simulink model "Modelo_global_NL_ley_de_control_minima_eje_d_q"  (R2023b)
settings: Solver=VariableStepAuto  StartTime=0.0  StopTime=1  RelTol=1e-3
values from neighbouring files (symbols this model uses):
  Ld = 6.6e-3    (= 0.0066)    [constantes.m]
  Lq = 5.8e-3    (= 0.0058)    [constantes.m]
  P_p = 3    [constantes.m]
settings Model: Creator=rodri  LastModifiedBy=nahue

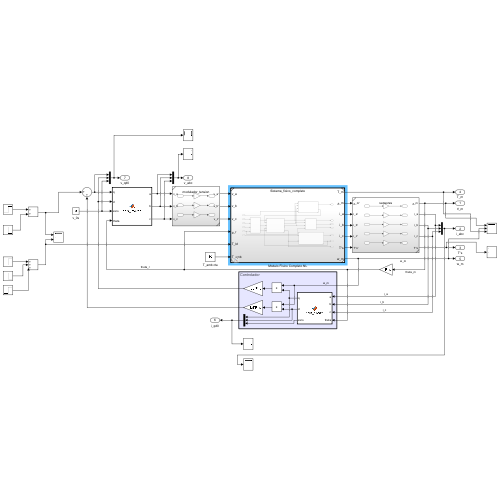
[thumbnail: Simulink's stored preview of the top-level diagram]
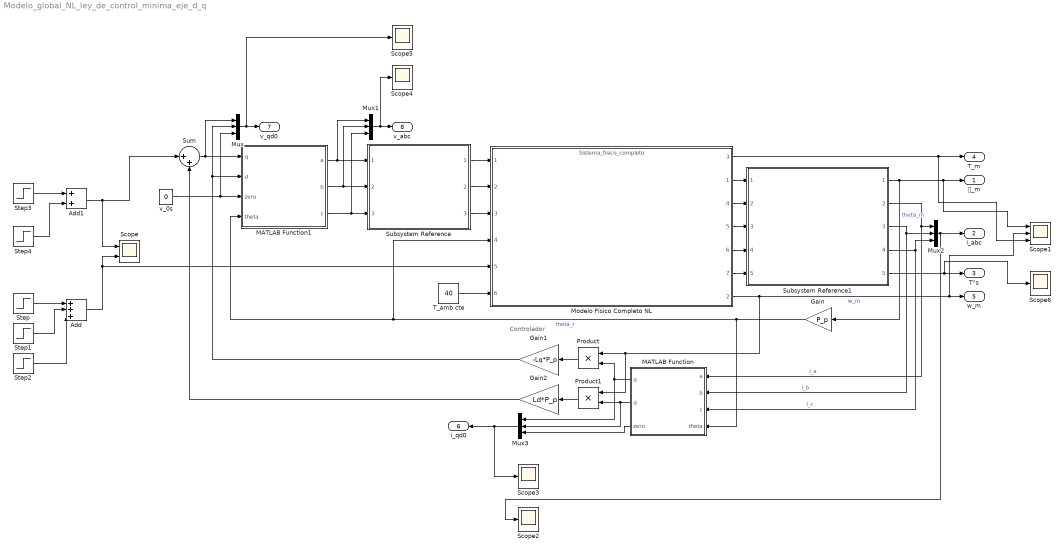
== system Modelo_global_NL_ley_de_control_minima_eje_d_q ==
  note: Controlador
  Add : Sum  Inputs=+++
  Add1 : Sum
  Gain : Gain  Gain=P_p
  Gain1 : Gain  Gain=-Lq*P_p
  Gain2 : Gain  Gain=Ld*P_p
  MATLAB Function : MATLAB Function  TreatAsAtomicUnit=on
  MATLAB Function1 : MATLAB Function  TreatAsAtomicUnit=on
  Modelo Físico Completo NL : ModelReference  ModelNameDialog=Sistema_fisico_completo.slx  SimulationMode=Normal  ModelReferenceVersion=1.15
      settings: PortSchema="{\"entries\":[{\"content\":{\"sides\":[{\"content\":{\"connectorIds\":[\"In1\",\"In2\",\"In3\",\"In4\",\"In5\",\"In6\"]},\"type\":\"ConnectorPlacement.EquallySpacedRectSide\",\"uuid\":\"c38844a2-9b74-4da6-b9ce-d4868a84fb83\"},{\"content\":{\"connectorIds\":[\"Out3\",\"Out1\",\"Out4\",\"Out5\",\"Out6\",\"Out7\",\"Out2\"],\"side\":\"RIGHT\"},\"type\":\"ConnectorPlacement.EquallySpacedRectSide\",\"uuid\":\"32cfc208-0644-4e1b-b9a9-83e6ff95cf9d\"},{\"content\":{\"side\":\"TOP\"},\"type\":\"ConnectorPlacement.EquallySpacedRectSide\",\"uuid\":\"4d8c9d59-309f-4ead-ae08-3f9c9c92e1b5\"}]},\"type\":\"ConnectorPlacement.EquallySpacedConnector\",\"uuid\":\"12663ecb-c0ca-4a2a-9423-b019766269d5\"}],\"packageUris\":[\"http://schema.mathworks.com/mf0/Connector/R2020b\"],\"version\":\"1.0\"}"
  Mux{,1..3} (4 alike) : Mux  Inputs=3
  Product : Product
  Product1 : Product
  Scope : Scope  NumInputPorts=2
  Scope1 : Scope  NumInputPorts=3
  Scope{2..6} (5 alike) : Scope
  Step : Step  Time=0.3  After=6.28  SampleTime=0.05
  Step1 : Step  Time=0.5  After=-6.28*2  SampleTime=0.05
  Step2 : Step  Time=0.9  After=6.28  SampleTime=0.05
  Step3 : Step  Time=0.1  After=19.596  SampleTime=0.05
  Step4 : Step  Time=0.7  After=-19.596  SampleTime=0.05
  Subsystem Reference : Subsystem  ReferencedSubsystem=modulador_tension
  Subsystem Reference1 : Subsystem  ReferencedSubsystem=sensores
  Sum : Sum  Inputs=|++
  T_amb cte : Constant  Value=40
  v_0s : Constant  Value=0
  𝜃_m : Outport
  i_abc : Outport  Port=2
  T°s : Outport  Port=3
  T_m : Outport  Port=4
  w_m : Outport  Port=5
  i_qd0 : Outport  Port=6
  v_qd0 : Outport  Port=7
  v_abc : Outport  Port=8
  wires:
  Subsystem Reference/1 -> Modelo Físico Completo NL/1
  Subsystem Reference/2 -> Modelo Físico Completo NL/2
  Subsystem Reference/3 -> Modelo Físico Completo NL/3
  Modelo Físico Completo NL/7 -> Subsystem Reference1/5
  Modelo Físico Completo NL/6 -> Subsystem Reference1/4
  Modelo Físico Completo NL/5 -> Subsystem Reference1/3
  Modelo Físico Completo NL/4 -> Subsystem Reference1/2
  Modelo Físico Completo NL/1 -> Subsystem Reference1/1
  v_0s/1 -> MATLAB Function1/3(zero), Mux/3
  MATLAB Function1/1(a) -> Mux1/1, Subsystem Reference/1
  MATLAB Function1/2(b) -> Mux1/2, Subsystem Reference/2
  MATLAB Function1/3(c) -> Mux1/3, Subsystem Reference/3
  T_amb cte/1 -> Modelo Físico Completo NL/6
  Subsystem Reference1/1 -> Gain/1, Scope1/1, 𝜃_m/1  "theta_m"
  Subsystem Reference1/2 -> Mux2/1, MATLAB Function/1(a)  "i_a"
  Subsystem Reference1/5 -> Scope6/1, T°s/1
  Subsystem Reference1/4 -> MATLAB Function/3(c), Mux2/3  "i_c"
  Subsystem Reference1/3 -> Mux2/2, MATLAB Function/2(b)  "i_b"
  Modelo Físico Completo NL/3 -> Scope1/3, T_m/1
  Gain/1 -> MATLAB Function/4(theta), Modelo Físico Completo NL/4, MATLAB Function1/4(theta)  "theta_r"
  Modelo Físico Completo NL/2 -> Product1/1, Product/1, Scope1/2, w_m/1  "w_m"
  MATLAB Function/1(q) -> Mux3/1, Product/2
  Product/1 -> Gain1/1
  Gain1/1 -> Mux/2, MATLAB Function1/2(d)
  MATLAB Function/2(d) -> Mux3/2, Product1/2
  MATLAB Function/3(zero) -> Mux3/3
  Mux/1 -> Scope5/1, v_qd0/1
  Mux1/1 -> Scope4/1, v_abc/1
  Mux2/1 -> Scope2/1, i_abc/1
  Mux3/1 -> Scope3/1, i_qd0/1
  Product1/1 -> Gain2/1
  Add1/1 -> Scope/1, Sum/1
  Sum/1 -> Mux/1, MATLAB Function1/1(q)
  Gain2/1 -> Sum/2
  Step/1 -> Add/1
  Step2/1 -> Add/3
  Step3/1 -> Add1/1
  Step1/1 -> Add/2
  Step4/1 -> Add1/2
  Add/1 -> Scope/2, Modelo Físico Completo NL/5

== matlab function Modelo_global_NL_ley_de_control_minima_eje_d_q/MATLAB Function1 ==
  data: q input; a output; d input; zero input; theta input; b output; c output
function [a, b, c] = park_inversa(q, d, zero, theta)
    % Transformación de Park Inversa
    % Entradas:
    %   d, q, z: Coordenadas en el marco rotatorio
    %   theta: Ángulo en radianes
    % Salidas:
    %   a, b, c: Valores trifásicos reconstruidos
    
    % Constantes
    alpha = 2 * pi / 3; % Desplazamiento angular entre fases
    
    % Cálculo de valores trifásicos
    a = q * cos(theta) + d * sin(theta) + zero;
    b = q * cos(theta - alpha) + d * sin(theta - alpha) + zero;
    c = q * cos(theta + alpha) + d * sin(theta + alpha) + zero;
end

== matlab function Modelo_global_NL_ley_de_control_minima_eje_d_q/MATLAB Function ==
  data: q output; a input; d output; b input; c input; theta input; zero output
function [q, d, zero] = park_directa(a, b, c, theta)
    % Transformación de Park Directa
    % Entradas:
    %   a, b, c: Valores trifásicos
    %   theta: Ángulo en radianes
    % Salidas:
    %   d, q, z: Coordenadas en el marco rotatorio
    
    % Constantes
    alpha = 2 * pi / 3; % Desplazamiento angular entre fases
    k = 2 / 3; % Escala para invarianza
    
    % Cálculo de coordenadas d, q, z
    q = k * (a * cos(theta) + b * cos(theta - alpha) + c * cos(theta + alpha));
    d = k * (a * sin(theta) + b * sin(theta - alpha) + c * sin(theta + alpha));
    zero = k * (a * 1/2 + b * 1/2 + c * 1/2);
end
